simulink model "refmodelsim"  (R2023a)
settings: Solver=ode23  StartTime=0.0  StopTime=10  RelTol=1e-6
values from neighbouring files (symbols this model uses):
  bp1 = NL1opt.BreakPoints    [adaptation_sim_part1.m]    (also in adaptation_sim_part2.m; refmodel.m = NL1{i}.BreakPoints)
  bp2 = NL2opt.BreakPoints    [adaptation_sim_part1.m]    (also in adaptation_sim_part2.m; refmodel.m = NL2{j}.BreakPoints)
  H = [1  1  0; 0.5  0  1]    [evaluations.mat]    (also in nonlinearities.mat; project.m = [  1,1,0)
  x0 = [1,1,1]    [adaptation_sim_part1.m]    (also in adaptation_sim_part2.m = [1,-1,1]; evaluations.m = [x01(a),x02(b),x03(c)]'; refmodel.m = [1,0,-0.6]; s_ts22.m = [])
settings Model: Creator=kwiktor  LastModifiedBy=kwiktor
settings DebuggingCC: UnconnectedInputMsg=warning  UnconnectedOutputMsg=warning  UnconnectedLineMsg=warning
settings ModelReferenceCC: EnableRefExpFcnMdlSchedulingChecks=on
settings RTWCC: DLArmComputeVersion=19.05

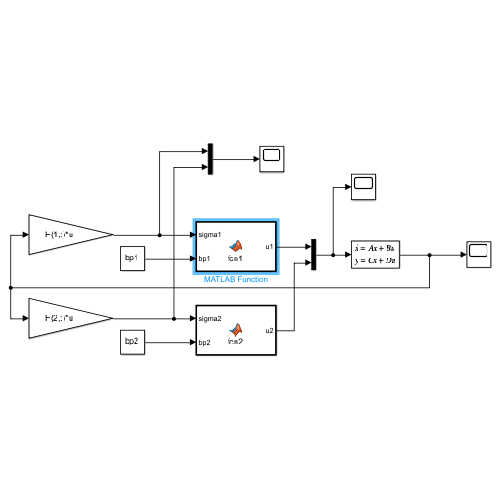
[thumbnail: Simulink's stored preview of the top-level diagram]
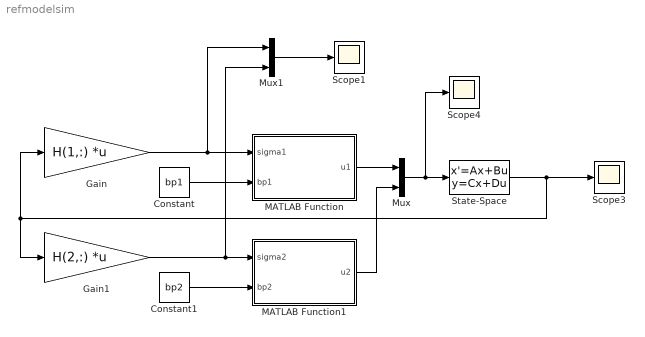
== system refmodelsim ==
  Constant : Constant  Value=bp1
  Constant1 : Constant  Value=bp2
  Gain : Gain  Gain=H(1,:)  Multiplication=Matrix(K*u)
  Gain1 : Gain  Gain=H(2,:)  Multiplication=Matrix(K*u)
  MATLAB Function : MATLAB Function  TreatAsAtomicUnit=on
  MATLAB Function1 : MATLAB Function  TreatAsAtomicUnit=on
  Mux : Mux  Inputs=2
  Mux1 : Mux  Inputs=2
  Scope1 : Scope
  Scope3 : Scope
  Scope4 : Scope
  State-Space : StateSpace  A=[-4,-9,-10; 1,0,0; 0,1,0]  B=[2,-1; 0,1; 1,0]  C=eye(3)  D=zeros(3,2)  InitialCondition=x0
  wires:
  State-Space/1 -> Gain/1, Gain1/1, Scope3/1
  Mux/1 -> Scope4/1, State-Space/1
  Gain/1 -> Mux1/1, MATLAB Function/1(sigma1)
  Gain1/1 -> Mux1/2, MATLAB Function1/1(sigma2)
  MATLAB Function1/1(u2) -> Mux/2
  MATLAB Function/1(u1) -> Mux/1
  Constant1/1 -> MATLAB Function1/2(bp2)
  Constant/1 -> MATLAB Function/2(bp1)
  Mux1/1 -> Scope1/1

== matlab function refmodelsim/MATLAB Function ==
  data: sigma1 input; u1 output; bp1 input
function u1 = fcn1(sigma1, bp1)

% linear controller
%u1 = bp1*sigma1;

% nonlinear controller
u1 = evaluatenl(bp1,sigma1);

== matlab function refmodelsim/MATLAB Function1 ==
  data: sigma2 input; u2 output; bp2 input
function u2 = fcn2(sigma2, bp2)

% linear controller
%u2 = bp2*sigma2;

% nonlinear controller
u2 = evaluatenl(bp2,sigma2);
